simulink model "Fusion_Frame_Model_Architecture"  (R2018a)
settings: Solver=FixedStepAuto  StartTime=0.0  StopTime=SimulationTime  FixedStep=SamplingTime  RelTol=1e-3
undefined symbols (not defined in the file or in its folder): ACTIVATE_CAM, ACTIVATE_RAD, CAM1_detTimeStamp, CAM1_MeasNoise, CAM1_objClassID, CAM1_PX, CAM1_PY, CAM1_VX, CAM1_VY, CAM2_detTimeStamp, CAM2_MeasNoise, CAM2_objClassID, CAM2_PX, CAM2_PY, CAM2_VX, CAM2_VY, CAM3_detTimeStamp, CAM3_MeasNoise, CAM3_objClassID, CAM3_PX, CAM3_PY, CAM3_VX, CAM3_VY, CAM4_detTimeStamp, CAM4_MeasNoise, CAM4_objClassID, CAM4_PX, CAM4_PY, CAM4_VX, CAM4_VY, CAM5_detTimeStamp, CAM5_MeasNoise, CAM5_objClassID, CAM5_PX, CAM5_PY, CAM5_VX, CAM5_VY, CAM6_detTimeStamp, CAM6_MeasNoise, CAM6_objClassID, CAM6_PX, CAM6_PY, CAM6_VX, CAM6_VY, CAM7_detTimeStamp, CAM7_MeasNoise, CAM7_objClassID, CAM7_PX, CAM7_PY, CAM7_VX, CAM7_VY, CAM8_detTimeStamp, CAM8_MeasNoise, CAM8_objClassID, CAM8_PX, CAM8_PY, CAM8_VX, CAM8_VY, CAM_nMeas, CAM_TYPE ... (+181)
libraries: simulink_extras x4
(part 11 of 11)

== system Fusion_Frame_Model_Architecture/SENSOR_FUSION_SYSTEM/OBJECT_TRACKER_SENSOR_FUSION/SENSOR_LAYOUT_AND_CHRACTERIZATION/PRE_COMPUTE_SENSOR_FOV_GRID/COMPUTE_CAMERA_SNSR_GRID/ComputeCoverageANDConfidence/Compute_Cell_X_and_Y_index/Compute_FOV_Overlap_with_Cell_and_Region_Confidence/If Action Subsystem/If Action Subsystem1 ==
  x : Inport
  y : Inport  Port=2
  Action Port : ActionPort  ActionType=then
  If Action Subsystem : Subsystem  TreatAsAtomicUnit=on
  If Action Subsystem1 : Subsystem  TreatAsAtomicUnit=on
  If Action Subsystem2 : Subsystem  TreatAsAtomicUnit=on
  If Action Subsystem3 : Subsystem  TreatAsAtomicUnit=on
  If Action Subsystem4 : Subsystem  TreatAsAtomicUnit=on
  If Action Subsystem5 : Subsystem  TreatAsAtomicUnit=on
  If Action Subsystem6 : Subsystem  TreatAsAtomicUnit=on
  If Action Subsystem7 : Subsystem  TreatAsAtomicUnit=on
  Subsystem2 : Subsystem
  Subsystem3 : Subsystem
  Subsystem4 : Subsystem
  RangeConfidence : Outport
  fovOverlap : Outport  Port=2
  wires:
  y/1 -> Subsystem2/1(y)
  x/1 -> Subsystem3/1(x)
  Subsystem2/1(y1) -> If Action Subsystem4/Action
  Subsystem3/3(x3) -> If Action Subsystem2/Action
  Subsystem3/2(x2) -> If Action Subsystem1/Action
  Subsystem2/3(y3) -> If Action Subsystem6/Action
  Subsystem3/4(x4) -> If Action Subsystem3/Action
  Subsystem2/4(y4) -> If Action Subsystem7/Action
  Subsystem2/2(y2) -> If Action Subsystem5/Action
  Subsystem3/1(x1) -> If Action Subsystem/Action
  If Action Subsystem/1(x1) -> Subsystem4/1(x1)
  If Action Subsystem1/1(x1) -> Subsystem4/2(x2)
  If Action Subsystem2/1(x1) -> Subsystem4/3(x3)
  If Action Subsystem3/1(x1) -> Subsystem4/4(x4)
  If Action Subsystem4/1(x1) -> Subsystem4/5(y1)
  If Action Subsystem5/1(x1) -> Subsystem4/6(y2)
  If Action Subsystem6/1(x1) -> Subsystem4/7(y3)
  If Action Subsystem7/1(x1) -> Subsystem4/8(y4)
  Subsystem4/1(RegionConfidence) -> RangeConfidence/1
  Subsystem4/2(FOVOverlap) -> fovOverlap/1

== system Fusion_Frame_Model_Architecture/SENSOR_FUSION_SYSTEM/OBJECT_TRACKER_SENSOR_FUSION/SENSOR_LAYOUT_AND_CHRACTERIZATION/PRE_COMPUTE_SENSOR_FOV_GRID/COMPUTE_CAMERA_SNSR_GRID/ComputeCoverageANDConfidence/Compute_Cell_X_and_Y_index/Compute_FOV_Overlap_with_Cell_and_Region_Confidence/If Action Subsystem/If Action Subsystem2 ==
  Action Port : ActionPort  ActionType=else
  Constant : Constant  Value=single(0)
  Constant1 : Constant  Value=false
  RegionConfidence : Outport
  fovOverlap : Outport  Port=2
  wires:
  Constant/1 -> RegionConfidence/1
  Constant1/1 -> fovOverlap/1

== system Fusion_Frame_Model_Architecture/SENSOR_FUSION_SYSTEM/OBJECT_TRACKER_SENSOR_FUSION/SENSOR_LAYOUT_AND_CHRACTERIZATION/PRE_COMPUTE_SENSOR_FOV_GRID/COMPUTE_RADAR_SNSR_GRID/ComputeCoverageANDConfidence/Compute_Cell_X_and_Y_index/Compute_FOV_Overlap_with_Cell_and_Region_Confidence/If Action Subsystem/Check_IF_Within_FOV ==
  Range : Inport
  In2 : Inport  Port=2
  SnsrIntrinsic : Inport  Port=3
  Abs : Abs
  Bus Selector : BusSelector  OutputSignals=MaxRange,MaxAzimuth
  GreaterThanOrEqual : RelationalOperator  Operator=<=  OutDataTypeStr=boolean  RndMeth=Simplest
  GreaterThanOrEqual1 : RelationalOperator  OutDataTypeStr=boolean  RndMeth=Simplest
  Logical Operator : Logic  AllPortsSameDT=off  OutDataTypeStr=boolean
  isWithinFOV : Outport
  wires:
  Bus Selector/1 -> GreaterThanOrEqual/2  "<MaxRange>"
  Logical Operator/1 -> isWithinFOV/1
  GreaterThanOrEqual/1 -> Logical Operator/1
  SnsrIntrinsic/1 -> Bus Selector/1
  Range/1 -> GreaterThanOrEqual/1
  GreaterThanOrEqual1/1 -> Logical Operator/2
  Bus Selector/2 -> GreaterThanOrEqual1/1  "<MaxAzimuth>"
  In2/1 -> Abs/1
  Abs/1 -> GreaterThanOrEqual1/2

== system Fusion_Frame_Model_Architecture/SENSOR_FUSION_SYSTEM/OBJECT_TRACKER_SENSOR_FUSION/SENSOR_LAYOUT_AND_CHRACTERIZATION/PRE_COMPUTE_SENSOR_FOV_GRID/COMPUTE_RADAR_SNSR_GRID/ComputeCoverageANDConfidence/Compute_Cell_X_and_Y_index/Compute_FOV_Overlap_with_Cell_and_Region_Confidence/If Action Subsystem/Compute_Range_Azimuth ==
  x : Inport
  y : Inport  Port=2
  Add : Sum
  Atan : Trigonometry  Operator=atan
  Divide : Product  Inputs=*/
  Radians to Degrees : simulink_extras/Transformations/Radians to Degrees
  Sqrt : Sqrt  SaturateOnIntegerOverflow=on
  Square : Math  Operator=square  SaturateOnIntegerOverflow=on
  Square1 : Math  Operator=square  SaturateOnIntegerOverflow=on
  Range : Outport
  Azimuth : Outport  Port=2
  wires:
  Square/1 -> Add/1
  Square1/1 -> Add/2
  Add/1 -> Sqrt/1
  Atan/1 -> Radians to Degrees/1
  Sqrt/1 -> Range/1
  Radians to Degrees/1 -> Azimuth/1
  Divide/1 -> Atan/1
  y/1 -> Square1/1, Divide/1
  x/1 -> Square/1, Divide/2

== system Fusion_Frame_Model_Architecture/SENSOR_FUSION_SYSTEM/OBJECT_TRACKER_SENSOR_FUSION/SENSOR_LAYOUT_AND_CHRACTERIZATION/PRE_COMPUTE_SENSOR_FOV_GRID/COMPUTE_RADAR_SNSR_GRID/ComputeCoverageANDConfidence/Compute_Cell_X_and_Y_index/Compute_FOV_Overlap_with_Cell_and_Region_Confidence/If Action Subsystem/If Action Subsystem1 ==
  x : Inport
  y : Inport  Port=2
  Action Port : ActionPort  ActionType=then
  If Action Subsystem : Subsystem  TreatAsAtomicUnit=on
  If Action Subsystem1 : Subsystem  TreatAsAtomicUnit=on
  If Action Subsystem2 : Subsystem  TreatAsAtomicUnit=on
  If Action Subsystem3 : Subsystem  TreatAsAtomicUnit=on
  If Action Subsystem4 : Subsystem  TreatAsAtomicUnit=on
  If Action Subsystem5 : Subsystem  TreatAsAtomicUnit=on
  If Action Subsystem6 : Subsystem  TreatAsAtomicUnit=on
  If Action Subsystem7 : Subsystem  TreatAsAtomicUnit=on
  Subsystem2 : Subsystem
  Subsystem3 : Subsystem
  Subsystem4 : Subsystem
  RangeConfidence : Outport
  fovOverlap : Outport  Port=2
  wires:
  y/1 -> Subsystem2/1(y)
  x/1 -> Subsystem3/1(x)
  Subsystem2/1(y1) -> If Action Subsystem4/Action
  Subsystem3/3(x3) -> If Action Subsystem2/Action
  Subsystem3/2(x2) -> If Action Subsystem1/Action
  Subsystem2/3(y3) -> If Action Subsystem6/Action
  Subsystem3/4(x4) -> If Action Subsystem3/Action
  Subsystem2/4(y4) -> If Action Subsystem7/Action
  Subsystem2/2(y2) -> If Action Subsystem5/Action
  Subsystem3/1(x1) -> If Action Subsystem/Action
  If Action Subsystem/1(x1) -> Subsystem4/1(x1)
  If Action Subsystem1/1(x1) -> Subsystem4/2(x2)
  If Action Subsystem2/1(x1) -> Subsystem4/3(x3)
  If Action Subsystem3/1(x1) -> Subsystem4/4(x4)
  If Action Subsystem4/1(x1) -> Subsystem4/5(y1)
  If Action Subsystem5/1(x1) -> Subsystem4/6(y2)
  If Action Subsystem6/1(x1) -> Subsystem4/7(y3)
  If Action Subsystem7/1(x1) -> Subsystem4/8(y4)
  Subsystem4/1(RegionConfidence) -> RangeConfidence/1
  Subsystem4/2(FOVOverlap) -> fovOverlap/1

== system Fusion_Frame_Model_Architecture/SENSOR_FUSION_SYSTEM/OBJECT_TRACKER_SENSOR_FUSION/SENSOR_LAYOUT_AND_CHRACTERIZATION/PRE_COMPUTE_SENSOR_FOV_GRID/COMPUTE_RADAR_SNSR_GRID/ComputeCoverageANDConfidence/Compute_Cell_X_and_Y_index/Compute_FOV_Overlap_with_Cell_and_Region_Confidence/If Action Subsystem/If Action Subsystem2 ==
  Action Port : ActionPort  ActionType=else
  Constant : Constant  Value=single(0)
  Constant1 : Constant  Value=false
  RegionConfidence : Outport
  fovOverlap : Outport  Port=2
  wires:
  Constant/1 -> RegionConfidence/1
  Constant1/1 -> fovOverlap/1

== system Fusion_Frame_Model_Architecture/SENSOR_FUSION_SYSTEM/OBJECT_TRACKER_SENSOR_FUSION/RADAR_HOMOGENEOUS_FUSION/SIMPLYFIED_DBSCAN_FOR_RADAR_MEASUREMENT_GROUPING/DBSCAN_MEASUREMENT_GROUPING/FORM_CLUSTER/DBSCAN/DBSCAN_PROPAGATE_AND_EXPAND_CLUSTER/EXPAND_CLUSTER/CLUSTER_EXPANSION/CHECK_CONDITION ==
  MEAS : Inport
  idx_i : Inport  Port=2
  idx_j : Inport  Port=3
  CLSTR_DATA_INIT : Inport  Port=4
  CLSTR_DATA_PREV : Inport  Port=5
  Bus Selector : BusSelector  OutputSignals=isMeasVisitedFlag
  Bus Selector1 : BusSelector  OutputSignals=MeasArray
  Constant2 : Constant  Value=dbscan_eps
  LessThanOrEqual1 : RelationalOperator  Operator=<=  OutDataTypeStr=boolean  RndMeth=Simplest
  Logical Operator : Logic  AllPortsSameDT=off  OutDataTypeStr=boolean
  Logical Operator1 : Logic  Operator=NOT  AllPortsSameDT=off  OutDataTypeStr=boolean
  Selector1 : Selector  NumberOfDimensions=2  InputPortWidth=3  IndexOptions=Select all,Index vector (port)  Indices=[1 3],1  OutputSizes=1,1
  Selector2 : Selector  NumberOfDimensions=2  InputPortWidth=3  IndexOptions=Select all,Index vector (port)  Indices=[1 3],1  OutputSizes=1,1
  Selector3 : Selector  NumberOfDimensions=2  InputPortWidth=3  IndexOptions=Select all,Index vector (port)  Indices=[1 3],1  OutputSizes=1,1
  Sqrt : Sqrt  SaturateOnIntegerOverflow=on
  Square : Math  Operator=square  SaturateOnIntegerOverflow=on
  Subtract : Sum  Inputs=+-
  Sum of Elements : Sum  Inputs=+
  Switch6 : Switch  Criteria=u2 > Threshold  Threshold=int32(1)
  Unit Delay : UnitDelay  InitialCondition=CLSTR_SNSR_DELAY_INIT  SampleTime=-1
  isMember : Outport
  CLSTR_DATA : Outport  Port=2
  wires:
  LessThanOrEqual1/1 -> Logical Operator/1
  Bus Selector/1 -> Selector1/1  "<isMeasVisitedFlag>"
  Logical Operator1/1 -> Logical Operator/2
  [x_i] -> Selector2/2
  Sqrt/1 -> LessThanOrEqual1/1
  idx_i/1 -> [x_i]
  Selector1/1 -> Logical Operator1/1
  idx_j/1 -> [y_j]
  [y_j] -> Selector3/2
  Selector3/1 -> Subtract/2
  Constant2/1 -> LessThanOrEqual1/2
  Selector2/1 -> Subtract/1
  Logical Operator/1 -> isMember/1
  [y_j] -> Selector1/2
  Subtract/1 -> Square/1
  MEAS/1 -> Bus Selector1/1
  Square/1 -> Sum of Elements/1
  Sum of Elements/1 -> Sqrt/1
  Unit Delay/1 -> Switch6/1
  [y_j] -> Switch6/2
  CLSTR_DATA_INIT/1 -> Switch6/3
  Switch6/1 -> CLSTR_DATA/1, Bus Selector/1
  CLSTR_DATA_PREV/1 -> Unit Delay/1
  Bus Selector1/1 -> Selector3/1, Selector2/1  "<MeasArray>"

== system Fusion_Frame_Model_Architecture/SENSOR_FUSION_SYSTEM/OBJECT_TRACKER_SENSOR_FUSION/RADAR_HOMOGENEOUS_FUSION/SIMPLYFIED_DBSCAN_FOR_RADAR_MEASUREMENT_GROUPING/DBSCAN_MEASUREMENT_GROUPING/FORM_CLUSTER/DBSCAN/DBSCAN_PROPAGATE_AND_EXPAND_CLUSTER/EXPAND_CLUSTER/CLUSTER_EXPANSION/SET_DATA ==
  isClusterMember : Inport
  CLSTR_DATA : Inport  Port=2
  idx_j : Inport  Port=3
  GET_DATA_FROM_BUS : Subsystem
  SET_CLUSTER_DATA_TO_BUS : Subsystem
  UPDATE_CLUSTER_DATA : Subsystem
  CLSTR_DATA_UPD : Outport
  wires:
  SET_CLUSTER_DATA_TO_BUS/1(CLSTR_DATA_UPD) -> CLSTR_DATA_UPD/1
  isClusterMember/1 -> UPDATE_CLUSTER_DATA/1(FLAG)
  idx_j/1 -> UPDATE_CLUSTER_DATA/2(idx_j)
  GET_DATA_FROM_BUS/1(<ClusterSizes>) -> UPDATE_CLUSTER_DATA/3(ClusterSizes)
  GET_DATA_FROM_BUS/2(<ClusterToMeasAssignment>) -> UPDATE_CLUSTER_DATA/4(Clstr2MeasAssign)
  GET_DATA_FROM_BUS/3(<isMeasVisitedFlag>) -> UPDATE_CLUSTER_DATA/5(MeasIsVisited)
  GET_DATA_FROM_BUS/4(<nClusters>) -> UPDATE_CLUSTER_DATA/6(nClusters)
  GET_DATA_FROM_BUS/5(<ClusterMember>) -> UPDATE_CLUSTER_DATA/7(ClstrMem)
  CLSTR_DATA/1 -> SET_CLUSTER_DATA_TO_BUS/5(CLSTR_DATA), GET_DATA_FROM_BUS/1(CLSTR_DATA)
  UPDATE_CLUSTER_DATA/1(isVisited) -> SET_CLUSTER_DATA_TO_BUS/1(isMeasVisitedFlag)
  UPDATE_CLUSTER_DATA/2(ClstrSize) -> SET_CLUSTER_DATA_TO_BUS/2(ClusterSizes)
  UPDATE_CLUSTER_DATA/3(ClstrAssignment) -> SET_CLUSTER_DATA_TO_BUS/3(ClusterToMeasAssignment)
  UPDATE_CLUSTER_DATA/4(ClstrMember) -> SET_CLUSTER_DATA_TO_BUS/4(ClusterMember)

== system Fusion_Frame_Model_Architecture/SENSOR_FUSION_SYSTEM/OBJECT_TRACKER_SENSOR_FUSION/SENSOR_LAYOUT_AND_CHRACTERIZATION/PRE_COMPUTE_SENSOR_FOV_GRID/COMPUTE_CAMERA_SNSR_GRID/ComputeCoverageANDConfidence/Compute_Cell_X_and_Y_index/Compute_FOV_Overlap_with_Cell_and_Region_Confidence/If Action Subsystem/If Action Subsystem1/If Action Subsystem ==
  Action Port : ActionPort  ActionType=then
  Constant : Constant  Value=int32(1)
  x1 : Outport
  wires:
  Constant/1 -> x1/1

== system Fusion_Frame_Model_Architecture/SENSOR_FUSION_SYSTEM/OBJECT_TRACKER_SENSOR_FUSION/SENSOR_LAYOUT_AND_CHRACTERIZATION/PRE_COMPUTE_SENSOR_FOV_GRID/COMPUTE_CAMERA_SNSR_GRID/ComputeCoverageANDConfidence/Compute_Cell_X_and_Y_index/Compute_FOV_Overlap_with_Cell_and_Region_Confidence/If Action Subsystem/If Action Subsystem1/If Action Subsystem1 ==
  Action Port : ActionPort  ActionType=elseif
  Constant : Constant  Value=int32(2)
  x1 : Outport
  wires:
  Constant/1 -> x1/1

== system Fusion_Frame_Model_Architecture/SENSOR_FUSION_SYSTEM/OBJECT_TRACKER_SENSOR_FUSION/SENSOR_LAYOUT_AND_CHRACTERIZATION/PRE_COMPUTE_SENSOR_FOV_GRID/COMPUTE_CAMERA_SNSR_GRID/ComputeCoverageANDConfidence/Compute_Cell_X_and_Y_index/Compute_FOV_Overlap_with_Cell_and_Region_Confidence/If Action Subsystem/If Action Subsystem1/If Action Subsystem2 ==
  Action Port : ActionPort  ActionType=elseif
  Constant : Constant  Value=int32(3)
  x1 : Outport
  wires:
  Constant/1 -> x1/1

== system Fusion_Frame_Model_Architecture/SENSOR_FUSION_SYSTEM/OBJECT_TRACKER_SENSOR_FUSION/SENSOR_LAYOUT_AND_CHRACTERIZATION/PRE_COMPUTE_SENSOR_FOV_GRID/COMPUTE_CAMERA_SNSR_GRID/ComputeCoverageANDConfidence/Compute_Cell_X_and_Y_index/Compute_FOV_Overlap_with_Cell_and_Region_Confidence/If Action Subsystem/If Action Subsystem1/If Action Subsystem3 ==
  Action Port : ActionPort  ActionType=elseif
  Constant : Constant  Value=int32(4)
  x1 : Outport
  wires:
  Constant/1 -> x1/1

== system Fusion_Frame_Model_Architecture/SENSOR_FUSION_SYSTEM/OBJECT_TRACKER_SENSOR_FUSION/SENSOR_LAYOUT_AND_CHRACTERIZATION/PRE_COMPUTE_SENSOR_FOV_GRID/COMPUTE_CAMERA_SNSR_GRID/ComputeCoverageANDConfidence/Compute_Cell_X_and_Y_index/Compute_FOV_Overlap_with_Cell_and_Region_Confidence/If Action Subsystem/If Action Subsystem1/If Action Subsystem4 ==
  Action Port : ActionPort  ActionType=then
  Constant : Constant  Value=int32(1)
  x1 : Outport
  wires:
  Constant/1 -> x1/1

== system Fusion_Frame_Model_Architecture/SENSOR_FUSION_SYSTEM/OBJECT_TRACKER_SENSOR_FUSION/SENSOR_LAYOUT_AND_CHRACTERIZATION/PRE_COMPUTE_SENSOR_FOV_GRID/COMPUTE_CAMERA_SNSR_GRID/ComputeCoverageANDConfidence/Compute_Cell_X_and_Y_index/Compute_FOV_Overlap_with_Cell_and_Region_Confidence/If Action Subsystem/If Action Subsystem1/If Action Subsystem5 ==
  Action Port : ActionPort  ActionType=elseif
  Constant : Constant  Value=int32(2)
  x1 : Outport
  wires:
  Constant/1 -> x1/1

== system Fusion_Frame_Model_Architecture/SENSOR_FUSION_SYSTEM/OBJECT_TRACKER_SENSOR_FUSION/SENSOR_LAYOUT_AND_CHRACTERIZATION/PRE_COMPUTE_SENSOR_FOV_GRID/COMPUTE_CAMERA_SNSR_GRID/ComputeCoverageANDConfidence/Compute_Cell_X_and_Y_index/Compute_FOV_Overlap_with_Cell_and_Region_Confidence/If Action Subsystem/If Action Subsystem1/If Action Subsystem6 ==
  Action Port : ActionPort  ActionType=elseif
  Constant : Constant  Value=int32(3)
  x1 : Outport
  wires:
  Constant/1 -> x1/1

== system Fusion_Frame_Model_Architecture/SENSOR_FUSION_SYSTEM/OBJECT_TRACKER_SENSOR_FUSION/SENSOR_LAYOUT_AND_CHRACTERIZATION/PRE_COMPUTE_SENSOR_FOV_GRID/COMPUTE_CAMERA_SNSR_GRID/ComputeCoverageANDConfidence/Compute_Cell_X_and_Y_index/Compute_FOV_Overlap_with_Cell_and_Region_Confidence/If Action Subsystem/If Action Subsystem1/If Action Subsystem7 ==
  Action Port : ActionPort  ActionType=elseif
  Constant : Constant  Value=int32(4)
  x1 : Outport
  wires:
  Constant/1 -> x1/1

== system Fusion_Frame_Model_Architecture/SENSOR_FUSION_SYSTEM/OBJECT_TRACKER_SENSOR_FUSION/SENSOR_LAYOUT_AND_CHRACTERIZATION/PRE_COMPUTE_SENSOR_FOV_GRID/COMPUTE_CAMERA_SNSR_GRID/ComputeCoverageANDConfidence/Compute_Cell_X_and_Y_index/Compute_FOV_Overlap_with_Cell_and_Region_Confidence/If Action Subsystem/If Action Subsystem1/Subsystem2 ==
  y : Inport
  Abs : Abs
  Constant3 : Constant  Value=CONFI_RANGE_Y
  GreaterThan10 : RelationalOperator  Operator=<=  OutDataTypeStr=boolean  RndMeth=Simplest
  GreaterThan11 : RelationalOperator  Operator=>  OutDataTypeStr=boolean  RndMeth=Simplest
  GreaterThan12 : RelationalOperator  Operator=<=  OutDataTypeStr=boolean  RndMeth=Simplest
  GreaterThan13 : RelationalOperator  Operator=>  OutDataTypeStr=boolean  RndMeth=Simplest
  GreaterThan7 : RelationalOperator  OutDataTypeStr=boolean  RndMeth=Simplest
  GreaterThan8 : RelationalOperator  Operator=<=  OutDataTypeStr=boolean  RndMeth=Simplest
  GreaterThan9 : RelationalOperator  Operator=>  OutDataTypeStr=boolean  RndMeth=Simplest
  If1 : If  NumInputs=4  IfExpression=u1 == 1  ElseIfExpressions=u2 == 1, u3 == 1, u4 == 1  ShowElse=off
  Logical Operator5 : Logic  AllPortsSameDT=off  OutDataTypeStr=boolean
  Logical Operator6 : Logic  AllPortsSameDT=off  OutDataTypeStr=boolean
  Logical Operator7 : Logic  AllPortsSameDT=off  OutDataTypeStr=boolean
  Reshape1 : Reshape  OutputDimensionality=Row vector (2-D)
  Selector4 : Selector  NumberOfDimensions=2  InputPortWidth=3  IndexOptions=Select all,Index vector (dialog)  Indices=[1 3],1  OutputSizes=1,1
  Selector5 : Selector  NumberOfDimensions=2  InputPortWidth=3  IndexOptions=Select all,Index vector (dialog)  Indices=[1 3],2  OutputSizes=1,1
  Selector6 : Selector  NumberOfDimensions=2  InputPortWidth=3  IndexOptions=Select all,Index vector (dialog)  Indices=[1 3],3  OutputSizes=1,1
  Selector7 : Selector  NumberOfDimensions=2  InputPortWidth=3  IndexOptions=Select all,Index vector (dialog)  Indices=[1 3],4  OutputSizes=1,1
  y1 : Outport
  y2 : Outport  Port=2
  y3 : Outport  Port=3
  y4 : Outport  Port=4
  wires:
  Selector4/1 -> [yLimit1]
  y/1 -> Abs/1
  [yLimit2] -> GreaterThan8/2
  If1/1 -> y1/1  "y1"
  Reshape1/1 -> Selector7/1, Selector6/1, Selector5/1, Selector4/1
  Logical Operator5/1 -> If1/1
  [yLimit2] -> GreaterThan9/2
  Logical Operator7/1 -> If1/3
  Selector5/1 -> [yLimit2]
  GreaterThan8/1 -> Logical Operator5/2
  [yLimit3] -> GreaterThan10/2
  GreaterThan13/1 -> If1/4
  Constant3/1 -> Reshape1/1
  [yLimit3] -> GreaterThan11/2
  If1/3 -> y3/1  "y3"
  Logical Operator6/1 -> If1/2
  GreaterThan10/1 -> Logical Operator6/2
  Selector7/1 -> [yLimit4]
  GreaterThan12/1 -> Logical Operator7/2
  Selector6/1 -> [yLimit3]
  GreaterThan7/1 -> Logical Operator5/1
  GreaterThan11/1 -> Logical Operator7/1
  [yLimit4] -> GreaterThan12/2
  [yLimit1] -> GreaterThan7/2
  If1/4 -> y4/1  "y4"
  [yLimit4] -> GreaterThan13/2
  GreaterThan9/1 -> Logical Operator6/1
  If1/2 -> y2/1  "y2"
  Abs/1 -> GreaterThan13/1, GreaterThan12/1, GreaterThan11/1, GreaterThan10/1, GreaterThan9/1, GreaterThan8/1, GreaterThan7/1

== system Fusion_Frame_Model_Architecture/SENSOR_FUSION_SYSTEM/OBJECT_TRACKER_SENSOR_FUSION/SENSOR_LAYOUT_AND_CHRACTERIZATION/PRE_COMPUTE_SENSOR_FOV_GRID/COMPUTE_CAMERA_SNSR_GRID/ComputeCoverageANDConfidence/Compute_Cell_X_and_Y_index/Compute_FOV_Overlap_with_Cell_and_Region_Confidence/If Action Subsystem/If Action Subsystem1/Subsystem3 ==
  x : Inport
  Constant2 : Constant  Value=CONFI_RANGE_X
  GreaterThan : RelationalOperator  OutDataTypeStr=boolean  RndMeth=Simplest
  GreaterThan1 : RelationalOperator  Operator=<=  OutDataTypeStr=boolean  RndMeth=Simplest
  GreaterThan2 : RelationalOperator  Operator=>  OutDataTypeStr=boolean  RndMeth=Simplest
  GreaterThan3 : RelationalOperator  Operator=<=  OutDataTypeStr=boolean  RndMeth=Simplest
  GreaterThan4 : RelationalOperator  Operator=>  OutDataTypeStr=boolean  RndMeth=Simplest
  GreaterThan5 : RelationalOperator  Operator=<=  OutDataTypeStr=boolean  RndMeth=Simplest
  GreaterThan6 : RelationalOperator  Operator=>  OutDataTypeStr=boolean  RndMeth=Simplest
  If : If  NumInputs=4  IfExpression=u1 == 1  ElseIfExpressions=u2 == 1, u3 == 1, u4 == 1  ShowElse=off
  Logical Operator : Logic  AllPortsSameDT=off  OutDataTypeStr=boolean
  Logical Operator3 : Logic  AllPortsSameDT=off  OutDataTypeStr=boolean
  Logical Operator4 : Logic  AllPortsSameDT=off  OutDataTypeStr=boolean
  Reshape : Reshape  OutputDimensionality=Row vector (2-D)
  Selector : Selector  NumberOfDimensions=2  InputPortWidth=3  IndexOptions=Select all,Index vector (dialog)  Indices=[1 3],1  OutputSizes=1,1
  Selector1 : Selector  NumberOfDimensions=2  InputPortWidth=3  IndexOptions=Select all,Index vector (dialog)  Indices=[1 3],2  OutputSizes=1,1
  Selector2 : Selector  NumberOfDimensions=2  InputPortWidth=3  IndexOptions=Select all,Index vector (dialog)  Indices=[1 3],3  OutputSizes=1,1
  Selector3 : Selector  NumberOfDimensions=2  InputPortWidth=3  IndexOptions=Select all,Index vector (dialog)  Indices=[1 3],4  OutputSizes=1,1
  x1 : Outport
  x2 : Outport  Port=2
  x3 : Outport  Port=3
  x4 : Outport  Port=4
  wires:
  Reshape/1 -> Selector3/1, Selector2/1, Selector1/1, Selector/1
  Logical Operator/1 -> If/1
  [xLimit2] -> GreaterThan1/2
  Logical Operator3/1 -> If/2
  x/1 -> GreaterThan6/1, GreaterThan5/1, GreaterThan4/1, GreaterThan3/1, GreaterThan2/1, GreaterThan1/1, GreaterThan/1
  Selector3/1 -> [xLimit4]
  GreaterThan4/1 -> Logical Operator4/1
  If/3 -> x3/1  "x3"
  GreaterThan6/1 -> If/4
  [xLimit1] -> GreaterThan/2
  [xLimit2] -> GreaterThan2/2
  Selector2/1 -> [xLimit3]
  [xLimit4] -> GreaterThan5/2
  GreaterThan5/1 -> Logical Operator4/2
  [xLimit4] -> GreaterThan6/2
  GreaterThan1/1 -> Logical Operator/2
  GreaterThan/1 -> Logical Operator/1
  Selector/1 -> [xLimit1]
  [xLimit3] -> GreaterThan3/2
  [xLimit3] -> GreaterThan4/2
  If/1 -> x1/1  "x1"
  GreaterThan2/1 -> Logical Operator3/1
  Selector1/1 -> [xLimit2]
  If/2 -> x2/1  "x2"
  If/4 -> x4/1  "x4"
  Constant2/1 -> Reshape/1
  Logical Operator4/1 -> If/3
  GreaterThan3/1 -> Logical Operator3/2

== system Fusion_Frame_Model_Architecture/SENSOR_FUSION_SYSTEM/OBJECT_TRACKER_SENSOR_FUSION/SENSOR_LAYOUT_AND_CHRACTERIZATION/PRE_COMPUTE_SENSOR_FOV_GRID/COMPUTE_CAMERA_SNSR_GRID/ComputeCoverageANDConfidence/Compute_Cell_X_and_Y_index/Compute_FOV_Overlap_with_Cell_and_Region_Confidence/If Action Subsystem/If Action Subsystem1/Subsystem4 ==
  x1 : Inport
  x2 : Inport  Port=2
  x3 : Inport  Port=3
  x4 : Inport  Port=4
  y1 : Inport  Port=5
  y2 : Inport  Port=6
  y3 : Inport  Port=7
  y4 : Inport  Port=8
  Constant1 : Constant  Value=true
  Constant2 : Constant  Value=CONFI_VALS
  Merge : Merge  Inputs=4
  Merge1 : Merge  Inputs=4
  Selector : Selector  NumberOfDimensions=2  InputPortWidth=3  IndexOptions=Index vector (port),Index vector (port)  Indices=[1 3],1  OutputSizes=1,1
  RegionConfidence : Outport
  FOVOverlap : Outport  Port=2
  wires:
  x2/1 -> Merge/2
  Constant1/1 -> FOVOverlap/1
  y4/1 -> Merge1/4
  Constant2/1 -> Selector/1
  y1/1 -> Merge1/1
  x1/1 -> Merge/1
  x4/1 -> Merge/4
  Selector/1 -> RegionConfidence/1
  y3/1 -> Merge1/3
  y2/1 -> Merge1/2
  x3/1 -> Merge/3
  Merge/1 -> Selector/2
  Merge1/1 -> Selector/3

== system Fusion_Frame_Model_Architecture/SENSOR_FUSION_SYSTEM/OBJECT_TRACKER_SENSOR_FUSION/SENSOR_LAYOUT_AND_CHRACTERIZATION/PRE_COMPUTE_SENSOR_FOV_GRID/COMPUTE_RADAR_SNSR_GRID/ComputeCoverageANDConfidence/Compute_Cell_X_and_Y_index/Compute_FOV_Overlap_with_Cell_and_Region_Confidence/If Action Subsystem/If Action Subsystem1/If Action Subsystem ==
  Action Port : ActionPort  ActionType=then
  Constant : Constant  Value=int32(1)
  x1 : Outport
  wires:
  Constant/1 -> x1/1

== system Fusion_Frame_Model_Architecture/SENSOR_FUSION_SYSTEM/OBJECT_TRACKER_SENSOR_FUSION/SENSOR_LAYOUT_AND_CHRACTERIZATION/PRE_COMPUTE_SENSOR_FOV_GRID/COMPUTE_RADAR_SNSR_GRID/ComputeCoverageANDConfidence/Compute_Cell_X_and_Y_index/Compute_FOV_Overlap_with_Cell_and_Region_Confidence/If Action Subsystem/If Action Subsystem1/If Action Subsystem1 ==
  Action Port : ActionPort  ActionType=elseif
  Constant : Constant  Value=int32(2)
  x1 : Outport
  wires:
  Constant/1 -> x1/1

== system Fusion_Frame_Model_Architecture/SENSOR_FUSION_SYSTEM/OBJECT_TRACKER_SENSOR_FUSION/SENSOR_LAYOUT_AND_CHRACTERIZATION/PRE_COMPUTE_SENSOR_FOV_GRID/COMPUTE_RADAR_SNSR_GRID/ComputeCoverageANDConfidence/Compute_Cell_X_and_Y_index/Compute_FOV_Overlap_with_Cell_and_Region_Confidence/If Action Subsystem/If Action Subsystem1/If Action Subsystem2 ==
  Action Port : ActionPort  ActionType=elseif
  Constant : Constant  Value=int32(3)
  x1 : Outport
  wires:
  Constant/1 -> x1/1

== system Fusion_Frame_Model_Architecture/SENSOR_FUSION_SYSTEM/OBJECT_TRACKER_SENSOR_FUSION/SENSOR_LAYOUT_AND_CHRACTERIZATION/PRE_COMPUTE_SENSOR_FOV_GRID/COMPUTE_RADAR_SNSR_GRID/ComputeCoverageANDConfidence/Compute_Cell_X_and_Y_index/Compute_FOV_Overlap_with_Cell_and_Region_Confidence/If Action Subsystem/If Action Subsystem1/If Action Subsystem3 ==
  Action Port : ActionPort  ActionType=elseif
  Constant : Constant  Value=int32(4)
  x1 : Outport
  wires:
  Constant/1 -> x1/1

== system Fusion_Frame_Model_Architecture/SENSOR_FUSION_SYSTEM/OBJECT_TRACKER_SENSOR_FUSION/SENSOR_LAYOUT_AND_CHRACTERIZATION/PRE_COMPUTE_SENSOR_FOV_GRID/COMPUTE_RADAR_SNSR_GRID/ComputeCoverageANDConfidence/Compute_Cell_X_and_Y_index/Compute_FOV_Overlap_with_Cell_and_Region_Confidence/If Action Subsystem/If Action Subsystem1/If Action Subsystem4 ==
  Action Port : ActionPort  ActionType=then
  Constant : Constant  Value=int32(1)
  x1 : Outport
  wires:
  Constant/1 -> x1/1

== system Fusion_Frame_Model_Architecture/SENSOR_FUSION_SYSTEM/OBJECT_TRACKER_SENSOR_FUSION/SENSOR_LAYOUT_AND_CHRACTERIZATION/PRE_COMPUTE_SENSOR_FOV_GRID/COMPUTE_RADAR_SNSR_GRID/ComputeCoverageANDConfidence/Compute_Cell_X_and_Y_index/Compute_FOV_Overlap_with_Cell_and_Region_Confidence/If Action Subsystem/If Action Subsystem1/If Action Subsystem5 ==
  Action Port : ActionPort  ActionType=elseif
  Constant : Constant  Value=int32(2)
  x1 : Outport
  wires:
  Constant/1 -> x1/1

== system Fusion_Frame_Model_Architecture/SENSOR_FUSION_SYSTEM/OBJECT_TRACKER_SENSOR_FUSION/SENSOR_LAYOUT_AND_CHRACTERIZATION/PRE_COMPUTE_SENSOR_FOV_GRID/COMPUTE_RADAR_SNSR_GRID/ComputeCoverageANDConfidence/Compute_Cell_X_and_Y_index/Compute_FOV_Overlap_with_Cell_and_Region_Confidence/If Action Subsystem/If Action Subsystem1/If Action Subsystem6 ==
  Action Port : ActionPort  ActionType=elseif
  Constant : Constant  Value=int32(3)
  x1 : Outport
  wires:
  Constant/1 -> x1/1

== system Fusion_Frame_Model_Architecture/SENSOR_FUSION_SYSTEM/OBJECT_TRACKER_SENSOR_FUSION/SENSOR_LAYOUT_AND_CHRACTERIZATION/PRE_COMPUTE_SENSOR_FOV_GRID/COMPUTE_RADAR_SNSR_GRID/ComputeCoverageANDConfidence/Compute_Cell_X_and_Y_index/Compute_FOV_Overlap_with_Cell_and_Region_Confidence/If Action Subsystem/If Action Subsystem1/If Action Subsystem7 ==
  Action Port : ActionPort  ActionType=elseif
  Constant : Constant  Value=int32(4)
  x1 : Outport
  wires:
  Constant/1 -> x1/1

== system Fusion_Frame_Model_Architecture/SENSOR_FUSION_SYSTEM/OBJECT_TRACKER_SENSOR_FUSION/SENSOR_LAYOUT_AND_CHRACTERIZATION/PRE_COMPUTE_SENSOR_FOV_GRID/COMPUTE_RADAR_SNSR_GRID/ComputeCoverageANDConfidence/Compute_Cell_X_and_Y_index/Compute_FOV_Overlap_with_Cell_and_Region_Confidence/If Action Subsystem/If Action Subsystem1/Subsystem2 ==
  y : Inport
  Abs : Abs
  Constant3 : Constant  Value=CONFI_RANGE_Y
  GreaterThan10 : RelationalOperator  Operator=<=  OutDataTypeStr=boolean  RndMeth=Simplest
  GreaterThan11 : RelationalOperator  Operator=>  OutDataTypeStr=boolean  RndMeth=Simplest
  GreaterThan12 : RelationalOperator  Operator=<=  OutDataTypeStr=boolean  RndMeth=Simplest
  GreaterThan13 : RelationalOperator  Operator=>  OutDataTypeStr=boolean  RndMeth=Simplest
  GreaterThan7 : RelationalOperator  OutDataTypeStr=boolean  RndMeth=Simplest
  GreaterThan8 : RelationalOperator  Operator=<=  OutDataTypeStr=boolean  RndMeth=Simplest
  GreaterThan9 : RelationalOperator  Operator=>  OutDataTypeStr=boolean  RndMeth=Simplest
  If1 : If  NumInputs=4  IfExpression=u1 == 1  ElseIfExpressions=u2 == 1, u3 == 1, u4 == 1  ShowElse=off
  Logical Operator5 : Logic  AllPortsSameDT=off  OutDataTypeStr=boolean
  Logical Operator6 : Logic  AllPortsSameDT=off  OutDataTypeStr=boolean
  Logical Operator7 : Logic  AllPortsSameDT=off  OutDataTypeStr=boolean
  Reshape1 : Reshape  OutputDimensionality=Row vector (2-D)
  Selector4 : Selector  NumberOfDimensions=2  InputPortWidth=3  IndexOptions=Select all,Index vector (dialog)  Indices=[1 3],1  OutputSizes=1,1
  Selector5 : Selector  NumberOfDimensions=2  InputPortWidth=3  IndexOptions=Select all,Index vector (dialog)  Indices=[1 3],2  OutputSizes=1,1
  Selector6 : Selector  NumberOfDimensions=2  InputPortWidth=3  IndexOptions=Select all,Index vector (dialog)  Indices=[1 3],3  OutputSizes=1,1
  Selector7 : Selector  NumberOfDimensions=2  InputPortWidth=3  IndexOptions=Select all,Index vector (dialog)  Indices=[1 3],4  OutputSizes=1,1
  y1 : Outport
  y2 : Outport  Port=2
  y3 : Outport  Port=3
  y4 : Outport  Port=4
  wires:
  Selector4/1 -> [yLimit1]
  y/1 -> Abs/1
  [yLimit2] -> GreaterThan8/2
  If1/1 -> y1/1  "y1"
  Reshape1/1 -> Selector7/1, Selector6/1, Selector5/1, Selector4/1
  Logical Operator5/1 -> If1/1
  [yLimit2] -> GreaterThan9/2
  Logical Operator7/1 -> If1/3
  Selector5/1 -> [yLimit2]
  GreaterThan8/1 -> Logical Operator5/2
  [yLimit3] -> GreaterThan10/2
  GreaterThan13/1 -> If1/4
  Constant3/1 -> Reshape1/1
  [yLimit3] -> GreaterThan11/2
  If1/3 -> y3/1  "y3"
  Logical Operator6/1 -> If1/2
  GreaterThan10/1 -> Logical Operator6/2
  Selector7/1 -> [yLimit4]
  GreaterThan12/1 -> Logical Operator7/2
  Selector6/1 -> [yLimit3]
  GreaterThan7/1 -> Logical Operator5/1
  GreaterThan11/1 -> Logical Operator7/1
  [yLimit4] -> GreaterThan12/2
  [yLimit1] -> GreaterThan7/2
  If1/4 -> y4/1  "y4"
  [yLimit4] -> GreaterThan13/2
  GreaterThan9/1 -> Logical Operator6/1
  If1/2 -> y2/1  "y2"
  Abs/1 -> GreaterThan13/1, GreaterThan12/1, GreaterThan11/1, GreaterThan10/1, GreaterThan9/1, GreaterThan8/1, GreaterThan7/1

== system Fusion_Frame_Model_Architecture/SENSOR_FUSION_SYSTEM/OBJECT_TRACKER_SENSOR_FUSION/SENSOR_LAYOUT_AND_CHRACTERIZATION/PRE_COMPUTE_SENSOR_FOV_GRID/COMPUTE_RADAR_SNSR_GRID/ComputeCoverageANDConfidence/Compute_Cell_X_and_Y_index/Compute_FOV_Overlap_with_Cell_and_Region_Confidence/If Action Subsystem/If Action Subsystem1/Subsystem3 ==
  x : Inport
  Constant2 : Constant  Value=CONFI_RANGE_X
  GreaterThan : RelationalOperator  OutDataTypeStr=boolean  RndMeth=Simplest
  GreaterThan1 : RelationalOperator  Operator=<=  OutDataTypeStr=boolean  RndMeth=Simplest
  GreaterThan2 : RelationalOperator  Operator=>  OutDataTypeStr=boolean  RndMeth=Simplest
  GreaterThan3 : RelationalOperator  Operator=<=  OutDataTypeStr=boolean  RndMeth=Simplest
  GreaterThan4 : RelationalOperator  Operator=>  OutDataTypeStr=boolean  RndMeth=Simplest
  GreaterThan5 : RelationalOperator  Operator=<=  OutDataTypeStr=boolean  RndMeth=Simplest
  GreaterThan6 : RelationalOperator  Operator=>  OutDataTypeStr=boolean  RndMeth=Simplest
  If : If  NumInputs=4  IfExpression=u1 == 1  ElseIfExpressions=u2 == 1, u3 == 1, u4 == 1  ShowElse=off
  Logical Operator : Logic  AllPortsSameDT=off  OutDataTypeStr=boolean
  Logical Operator3 : Logic  AllPortsSameDT=off  OutDataTypeStr=boolean
  Logical Operator4 : Logic  AllPortsSameDT=off  OutDataTypeStr=boolean
  Reshape : Reshape  OutputDimensionality=Row vector (2-D)
  Selector : Selector  NumberOfDimensions=2  InputPortWidth=3  IndexOptions=Select all,Index vector (dialog)  Indices=[1 3],1  OutputSizes=1,1
  Selector1 : Selector  NumberOfDimensions=2  InputPortWidth=3  IndexOptions=Select all,Index vector (dialog)  Indices=[1 3],2  OutputSizes=1,1
  Selector2 : Selector  NumberOfDimensions=2  InputPortWidth=3  IndexOptions=Select all,Index vector (dialog)  Indices=[1 3],3  OutputSizes=1,1
  Selector3 : Selector  NumberOfDimensions=2  InputPortWidth=3  IndexOptions=Select all,Index vector (dialog)  Indices=[1 3],4  OutputSizes=1,1
  x1 : Outport
  x2 : Outport  Port=2
  x3 : Outport  Port=3
  x4 : Outport  Port=4
  wires:
  Reshape/1 -> Selector3/1, Selector2/1, Selector1/1, Selector/1
  Logical Operator/1 -> If/1
  [xLimit2] -> GreaterThan1/2
  Logical Operator3/1 -> If/2
  x/1 -> GreaterThan6/1, GreaterThan5/1, GreaterThan4/1, GreaterThan3/1, GreaterThan2/1, GreaterThan1/1, GreaterThan/1
  Selector3/1 -> [xLimit4]
  GreaterThan4/1 -> Logical Operator4/1
  If/3 -> x3/1  "x3"
  GreaterThan6/1 -> If/4
  [xLimit1] -> GreaterThan/2
  [xLimit2] -> GreaterThan2/2
  Selector2/1 -> [xLimit3]
  [xLimit4] -> GreaterThan5/2
  GreaterThan5/1 -> Logical Operator4/2
  [xLimit4] -> GreaterThan6/2
  GreaterThan1/1 -> Logical Operator/2
  GreaterThan/1 -> Logical Operator/1
  Selector/1 -> [xLimit1]
  [xLimit3] -> GreaterThan3/2
  [xLimit3] -> GreaterThan4/2
  If/1 -> x1/1  "x1"
  GreaterThan2/1 -> Logical Operator3/1
  Selector1/1 -> [xLimit2]
  If/2 -> x2/1  "x2"
  If/4 -> x4/1  "x4"
  Constant2/1 -> Reshape/1
  Logical Operator4/1 -> If/3
  GreaterThan3/1 -> Logical Operator3/2

== system Fusion_Frame_Model_Architecture/SENSOR_FUSION_SYSTEM/OBJECT_TRACKER_SENSOR_FUSION/SENSOR_LAYOUT_AND_CHRACTERIZATION/PRE_COMPUTE_SENSOR_FOV_GRID/COMPUTE_RADAR_SNSR_GRID/ComputeCoverageANDConfidence/Compute_Cell_X_and_Y_index/Compute_FOV_Overlap_with_Cell_and_Region_Confidence/If Action Subsystem/If Action Subsystem1/Subsystem4 ==
  x1 : Inport
  x2 : Inport  Port=2
  x3 : Inport  Port=3
  x4 : Inport  Port=4
  y1 : Inport  Port=5
  y2 : Inport  Port=6
  y3 : Inport  Port=7
  y4 : Inport  Port=8
  Constant1 : Constant  Value=true
  Constant2 : Constant  Value=CONFI_VALS
  Merge : Merge  Inputs=4
  Merge1 : Merge  Inputs=4
  Selector : Selector  NumberOfDimensions=2  InputPortWidth=3  IndexOptions=Index vector (port),Index vector (port)  Indices=[1 3],1  OutputSizes=1,1
  RegionConfidence : Outport
  FOVOverlap : Outport  Port=2
  wires:
  x2/1 -> Merge/2
  Constant1/1 -> FOVOverlap/1
  y4/1 -> Merge1/4
  Constant2/1 -> Selector/1
  y1/1 -> Merge1/1
  x1/1 -> Merge/1
  x4/1 -> Merge/4
  Selector/1 -> RegionConfidence/1
  y3/1 -> Merge1/3
  y2/1 -> Merge1/2
  x3/1 -> Merge/3
  Merge/1 -> Selector/2
  Merge1/1 -> Selector/3

== system Fusion_Frame_Model_Architecture/SENSOR_FUSION_SYSTEM/OBJECT_TRACKER_SENSOR_FUSION/RADAR_HOMOGENEOUS_FUSION/SIMPLYFIED_DBSCAN_FOR_RADAR_MEASUREMENT_GROUPING/DBSCAN_MEASUREMENT_GROUPING/FORM_CLUSTER/DBSCAN/DBSCAN_PROPAGATE_AND_EXPAND_CLUSTER/EXPAND_CLUSTER/CLUSTER_EXPANSION/SET_DATA/GET_DATA_FROM_BUS ==
  CLSTR_DATA : Inport
  Bus Selector : BusSelector  OutputSignals=ClusterSizes,ClusterToMeasAssignment,isMeasVisitedFlag,nClusters,ClusterMember
  <ClusterSizes> : Outport
  <ClusterToMeasAssignment> : Outport  Port=2
  <isMeasVisitedFlag> : Outport  Port=3
  <nClusters> : Outport  Port=4
  <ClusterMember> : Outport  Port=5
  wires:
  CLSTR_DATA/1 -> Bus Selector/1
  Bus Selector/2 -> <ClusterToMeasAssignment>/1  "<ClusterToMeasAssignment>"
  Bus Selector/3 -> <isMeasVisitedFlag>/1  "<isMeasVisitedFlag>"
  Bus Selector/5 -> <ClusterMember>/1  "<ClusterMember>"
  Bus Selector/1 -> <ClusterSizes>/1  "<ClusterSizes>"
  Bus Selector/4 -> <nClusters>/1  "<nClusters>"

== system Fusion_Frame_Model_Architecture/SENSOR_FUSION_SYSTEM/OBJECT_TRACKER_SENSOR_FUSION/RADAR_HOMOGENEOUS_FUSION/SIMPLYFIED_DBSCAN_FOR_RADAR_MEASUREMENT_GROUPING/DBSCAN_MEASUREMENT_GROUPING/FORM_CLUSTER/DBSCAN/DBSCAN_PROPAGATE_AND_EXPAND_CLUSTER/EXPAND_CLUSTER/CLUSTER_EXPANSION/SET_DATA/SET_CLUSTER_DATA_TO_BUS ==
  isMeasVisitedFlag : Inport
  ClusterSizes : Inport  Port=2
  ClusterToMeasAssignment : Inport  Port=3
  ClusterMember : Inport  Port=4
  CLSTR_DATA : Inport  Port=5
  Bus Creator : BusCreator  Inputs=7  OutDataTypeStr=Bus: CLUSTER_DATA_STRUCT_SNSR  NonVirtualBus=on
      settings: InheritFromInputs=off
  Bus Selector1 : BusSelector  OutputSignals=ClusterCenter,ClusterCovariance,ClusterSizes,ClusterToMeasAssignment,isMeasVisitedFlag,nClusters,ClusterMember
  Terminator{,1..2,4} (4 alike) : Terminator
  CLSTR_DATA_UPD : Outport
  wires:
  Bus Selector1/6 -> Bus Creator/6  "<nClusters>"
  Bus Selector1/1 -> Bus Creator/1  "<ClusterCenter>"
  Bus Selector1/2 -> Bus Creator/2  "<ClusterCovariance>"
  Bus Selector1/4 -> Terminator2/1  "<ClusterToMeasAssignment>"
  Bus Selector1/7 -> Terminator4/1  "<ClusterMember>"
  Bus Selector1/5 -> Terminator/1  "<isMeasVisitedFlag>"
  Bus Selector1/3 -> Terminator1/1  "<ClusterSizes>"
  CLSTR_DATA/1 -> Bus Selector1/1
  Bus Creator/1 -> CLSTR_DATA_UPD/1
  ClusterToMeasAssignment/1 -> Bus Creator/4  "ClusterToMeasAssignment"
  isMeasVisitedFlag/1 -> Bus Creator/5  "isMeasVisitedFlag"
  ClusterMember/1 -> Bus Creator/7  "ClusterMember"
  ClusterSizes/1 -> Bus Creator/3  "ClusterSizes"

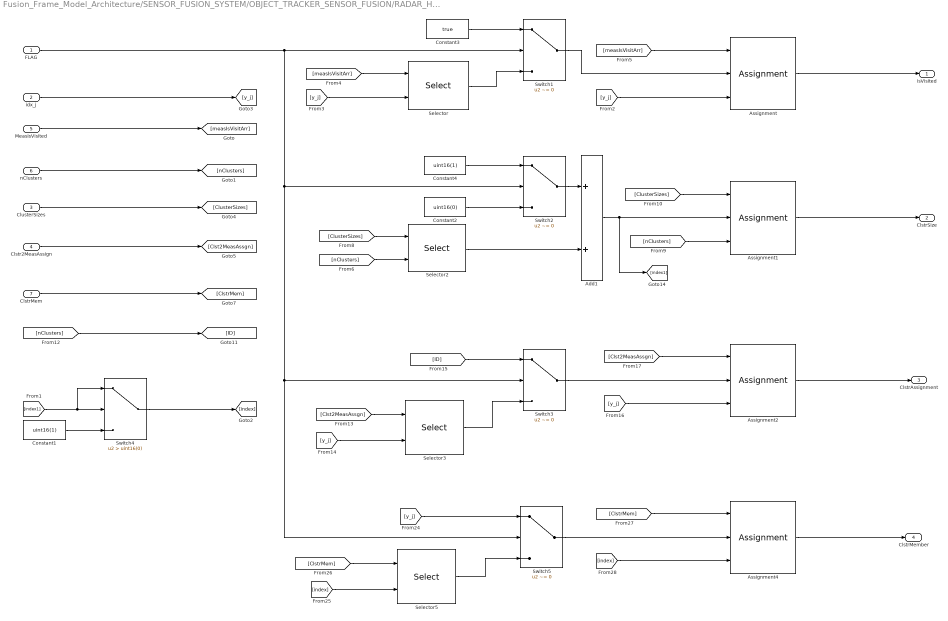
== system Fusion_Frame_Model_Architecture/SENSOR_FUSION_SYSTEM/OBJECT_TRACKER_SENSOR_FUSION/RADAR_HOMOGENEOUS_FUSION/SIMPLYFIED_DBSCAN_FOR_RADAR_MEASUREMENT_GROUPING/DBSCAN_MEASUREMENT_GROUPING/FORM_CLUSTER/DBSCAN/DBSCAN_PROPAGATE_AND_EXPAND_CLUSTER/EXPAND_CLUSTER/CLUSTER_EXPANSION/SET_DATA/UPDATE_CLUSTER_DATA ==
  FLAG : Inport
  idx_j : Inport  Port=2
  ClusterSizes : Inport  Port=3
  Clstr2MeasAssign : Inport  Port=4
  MeasIsVisited : Inport  Port=5
  nClusters : Inport  Port=6
  ClstrMem : Inport  Port=7
  Add1 : Sum
  Assignment{,1..2,4} (4 alike) : Assignment  NumberOfDimensions=2  DiagnosticForDimensions=Warning  IndexOptions=Assign all,Index vector (port)  Indices=1,1  OutputSizes=1,1
  Constant1 : Constant  Value=uint16(1)
  Constant2 : Constant  Value=uint16(0)
  Constant3 : Constant  Value=true
  Constant4 : Constant  Value=uint16(1)
  Selector{,2..3,5} (4 alike) : Selector  NumberOfDimensions=2  InputPortWidth=3  IndexOptions=Select all,Index vector (port)  Indices=[1 3],1  OutputSizes=1,1
  Switch{1..3,5} (4 alike) : Switch  Criteria=u2 ~= 0
  Switch4 : Switch  Criteria=u2 > Threshold  Threshold=uint16(0)
  isVisited : Outport
  ClstrSize : Outport  Port=2
  ClstrAssignment : Outport  Port=3
  ClstrMember : Outport  Port=4
  wires:
  [ClusterSizes] -> Assignment1/1
  [y_j] -> Selector3/2
  Switch1/1 -> Assignment/2
  [y_j] -> Assignment/3
  [ID] -> Switch3/1
  FLAG/1 -> Switch1/2, Switch5/2, Switch3/2, Switch2/2
  Assignment4/1 -> ClstrMember/1
  Selector3/1 -> Switch3/3
  Selector/1 -> Switch1/3
  [ClusterSizes] -> Selector2/1
  [Clst2MeasAssgn] -> Assignment2/1
  Constant3/1 -> Switch1/1
  Assignment/1 -> isVisited/1
  Switch5/1 -> Assignment4/2
  [ClstrMem] -> Selector5/1
  [measIsVisitArr] -> Assignment/1
  [y_j] -> Selector/2
  [y_j] -> Switch5/1
  [measIsVisitArr] -> Selector/1
  [nClusters] -> [ID]
  Add1/1 -> Assignment1/2, [index1]
  [nClusters] -> Assignment1/3
  Constant4/1 -> Switch2/1
  Constant2/1 -> Switch2/3
  [index] -> Assignment4/3
  [ClstrMem] -> Assignment4/1
  Assignment1/1 -> ClstrSize/1
  Selector5/1 -> Switch5/3
  Switch3/1 -> Assignment2/2
  Selector2/1 -> Add1/2
  [Clst2MeasAssgn] -> Selector3/1
  Switch2/1 -> Add1/1
  Assignment2/1 -> ClstrAssignment/1
  [index] -> Selector5/2
  [nClusters] -> Selector2/2
  [y_j] -> Assignment2/3
  idx_j/1 -> [y_j]
  MeasIsVisited/1 -> [measIsVisitArr]
  nClusters/1 -> [nClusters]
  ClusterSizes/1 -> [ClusterSizes]
  Clstr2MeasAssign/1 -> [Clst2MeasAssgn]
  ClstrMem/1 -> [ClstrMem]
  [index1] -> Switch4/1, Switch4/2
  Constant1/1 -> Switch4/3
  Switch4/1 -> [index]

== matlab function Fusion_Frame_Model_Architecture/SENSOR_FUSION_SYSTEM/OBJECT_TRACKER_SENSOR_FUSION/RADAR_HOMOGENEOUS_FUSION/GATING/MEASUREMENT_TO_TRACK_GATING_AND_LOGLIKELIHOOD_COMPUTATION/GATE_MEASUREMENTS_AND_COMPUTE_LIKELIHOOD/MAHALANOBIS_DISTANCE/MATLAB Function ==
  data: InnoCov input; InnoCovInverse output
function InnoCovInverse = fcn(InnoCov)
         InnoCovInverse = 1./InnoCov;
end

== matlab function Fusion_Frame_Model_Architecture/SENSOR_FUSION_SYSTEM/OBJECT_TRACKER_SENSOR_FUSION/RADAR_HOMOGENEOUS_FUSION/GATING/MEASUREMENT_TO_TRACK_GATING_AND_LOGLIKELIHOOD_COMPUTATION/GATE_MEASUREMENTS_AND_COMPUTE_LIKELIHOOD/GATE_MEASUREMENT_AND_COMPUTE_LOG_LIKELIHOOD/MATLAB Function1 ==
  data: InnoCov input; detInnoCov output
function detInnoCov  = ComputeDeterminant(InnoCov)
detInnoCov = det(InnoCov);
end

== matlab function Fusion_Frame_Model_Architecture/SENSOR_FUSION_SYSTEM/OBJECT_TRACKER_SENSOR_FUSION/RADAR_HOMOGENEOUS_FUSION/SEGREGATE_CLUSTER/MATLAB Function ==
  data: SENSORMeasCTS input; MeasArray output; SENSOR_CLUSTERS input; MeasCovariance output; ClusterRef output; ValidMeasCount output; ValidCumulativeMeasCount output
function [MeasArray, MeasCovariance, ClusterRef, ValidMeasCount, ValidCumulativeMeasCount] = SEGREGATE_CLUSTER(SENSORMeasCTS, SENSOR_CLUSTERS)
     
    nSensors = length(SENSORMeasCTS.ValidCumulativeMeasCount); % total number of sensors installed around the ego vehicle
    nMeas = SENSORMeasCTS.ValidCumulativeMeasCount(end);       % total number of measurements received  
    nSnsrClsters = SENSOR_CLUSTERS.nClusters;                  % total number of measurement clusters (all radars combined)
    countTotal = int16(0);
            
    % Initializations for the output
    MeasArray = single(zeros(2 , 1200));
    MeasCovariance = single(zeros(2, 2, 1200));
    ClusterRef = uint16(zeros(2 , 1200));
    ValidMeasCount = uint16(zeros(1,6));
    x = single(zeros(2,1)); R = single(zeros(2,2)); xSpread = single(zeros(2,2));
            
    for snsrIdx = 1:nSensors            % iterate over each of the sensors
        for idxClstr = 1:nSnsrClsters   % for each of the Radar clusters
            % 1. extract the associated cluster IDs
            clusterID = uint16(idxClstr); 
            % 2. extract the measurement IDs forming the cluster
            measIDsIndex = find(clusterID == SENSOR_CLUSTERS.ClusterToMeasAssignment(1,1:nMeas)); 
            % 3. extract the associated measurement IDs for each of the sensors
            measIDs = measIDsIndex(snsrIdx == SENSORMeasCTS.MeasRef(2,measIDsIndex)); 
            if(~isempty(measIDs))
               countTotal = countTotal + 1;
               weight = 1/length(measIDs);
               x(:) = 0; R(:) = 0;xSpread(:) = 0;
               for idxMeas = 1:length(measIDs)   % for each of the extracted measurements compute the weighted mean and covariance
                   x = x + weight.*SENSORMeasCTS.MeasArray(:,measIDs(idxMeas));
                   R = R + weight.*SENSORMeasCTS.MeasCovariance(:,:,measIDs(idxMeas));
               end
               for idxMeas = 1:length(measIDs)   % compute the spread of the mean
                   z = SENSORMeasCTS.MeasArray(:,measIDs(idxMeas));
                   xSpread = xSpread + weight.*( (x - z)*(x - z)' );
               end
               %R = R + xSpread;
               MeasArray(:,countTotal) = x;
               MeasCovariance(:,:,countTotal) = R;
               ClusterRef(1,countTotal) = snsrIdx;
               ClusterRef(2,countTotal) = clusterID;
               ValidMeasCount(1,snsrIdx) = ValidMeasCount(1,snsrIdx) + 1;
            end
        end
    end
    ValidCumulativeMeasCount = cumsum(ValidMeasCount);
end
